simulink model "labcartpid_new"  (Simulink 10.2)
settings: Solver=FixedStepAuto  StartTime=0.0  StopTime=29  FixedStep=0.001  RelTol=1e-3
values from neighbouring files (symbols this model uses):
  X_MAX = 0.6    [5.1wksp_1.mat]
undefined symbols (not defined in the file or in its folder): HIL, qc_get_step_size
libraries: quarc_library x5, simulink_need_slupdate x1, simulink x1
settings Model: Creator=pcadm  LastModifiedBy=pcadm  ExtModeTrigDuration=15000
settings SolverCC: PositivePriorityOrder=on
settings DataIOCC: SaveFormat=Dataset  SignalLoggingSaveFormat=Dataset
settings DebuggingCC: UnderspecifiedInitializationDetection=Simplified  MergeDetectMultiDrivingBlocksExec=error  FcnCallInpInsideContextMsg=error  SFUnexpectedBacktrackingDiag=error  SFNoUnconditionalDefaultTransitionDiag=error  SFExecutionAtInitializationDiag=warning
settings HardwareCC: ProdBitPerPointer=64  ProdBitPerSizeT=64  ProdBitPerPtrDiffT=64  ProdLargestAtomicFloat=Float  ProdIntDivRoundTo=Zero  ProdEndianess=LittleEndian  ProdWordSize=64  ProdHWDeviceType=Intel->x86-64 (Windows64)
settings ModelReferenceCC: PropagateSignalLabelsOutOfModel=on
settings RTWCC: Description=QUARC Win64 Target  SystemTargetFile=quarc_win64.tlc  TemplateMakefile=quarc_default_tmf
settings STFCustomTargetCC: TargetPreCompLibLocation=C:\PROGRA~3\QUARC\lib\2020b\win64\release  TargetLangStandard=C99 (ISO)  ConcurrentExecutionCompliant=on  SystemTargetFile=quarc_win64.tlc
settings GRTTargetCC: TargetPreCompLibLocation=C:\PROGRA~3\QUARC\lib\2020b\win64\release  TargetLangStandard=C99 (ISO)  ParMdlRefBuildCompliant=off  CompOptLevelCompliant=off  MatFileLogging=off  CPPClassGenCompliant=off  UseToolchainInfoCompliant=off  ExtMode=on  ExtModeMexFile=quarc_comm
settings ConfigComp: CovMetricSettings=dswe  CovSaveCumulativeToWorkspaceVar=off  CovSaveSingleToWorkspaceVar=off  CovExternalEMLEnable=on

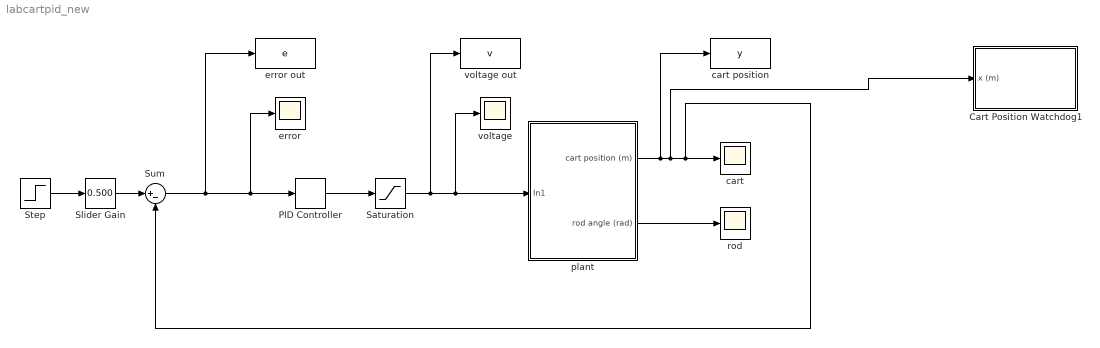
== system labcartpid_new ==
  Cart Position Watchdog1 : Subsystem  TreatAsAtomicUnit=on
  PID Controller : simulink_need_slupdate/PID Controller  P=80  I=2  D=10
  Saturation : Saturate  UpperLimit=6  LowerLimit=-6
  Slider Gain : simulink/Math Operations/Slider Gain  gain=0.500  low=-0.2  high=0.5
  Step : Step  Time=0  After=1.0  SampleTime=0
  Sum : Sum  Inputs=|+-
  cart : Scope
  cart position : ToWorkspace  VariableName=y  SaveFormat=Structure With Time  SampleTime=-1
  error : Scope
  error out : ToWorkspace  VariableName=e  SaveFormat=Structure  SampleTime=-1
  plant : Subsystem
  rod : Scope
  voltage : Scope
  voltage out : ToWorkspace  VariableName=v  SaveFormat=Structure  SampleTime=-1
  wires:
  Slider Gain/1 -> Sum/1
  Saturation/1 -> voltage out/1, plant/1(In1), voltage/1
  PID Controller/1 -> Saturation/1
  Sum/1 -> error/1, PID Controller/1, error out/1
  plant/1(cart position (m)) -> cart position/1, Cart Position Watchdog1/1(x (m)), cart/1, Sum/2
  Step/1 -> Slider Gain/1
  plant/2(rod angle (rad)) -> rod/1

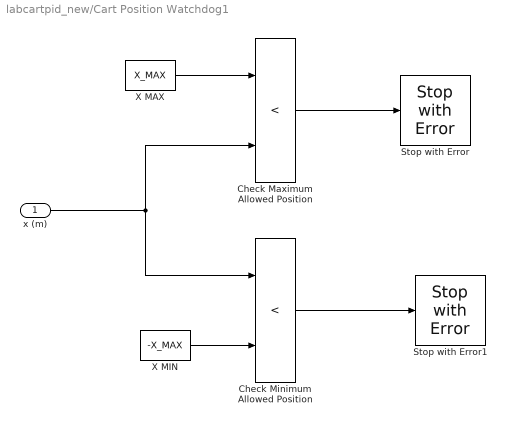
== system labcartpid_new/Cart Position Watchdog1 ==
  x (m) : Inport
  Check Maximum Allowed Position : RelationalOperator  Operator=<  RndMeth=Nearest  InputSameDT=on
  Check Minimum Allowed Position : RelationalOperator  Operator=<  RndMeth=Nearest  InputSameDT=on
  Stop with Error : quarc_library/Sinks/Error Handling/Stop with Error  message_type=Fixed error message  message=Maximum Limit Reached
      settings: AttributesFormatString="\"%<message>\""  SourceProductName=QUARC Targets
  Stop with Error1 : quarc_library/Sinks/Error Handling/Stop with Error  message_type=Fixed error message  message=Minimum Limit Reached
      settings: AttributesFormatString="\"%<message>\""  SourceProductName=QUARC Targets
  X MAX : Constant  Value=X_MAX
  X MIN : Constant  Value=-X_MAX
  wires:
  Check Maximum Allowed Position/1 -> Stop with Error/1
  x (m)/1 -> Check Minimum Allowed Position/1, Check Maximum Allowed Position/2
  X MIN/1 -> Check Minimum Allowed Position/2
  Check Minimum Allowed Position/1 -> Stop with Error1/1
  X MAX/1 -> Check Maximum Allowed Position/1

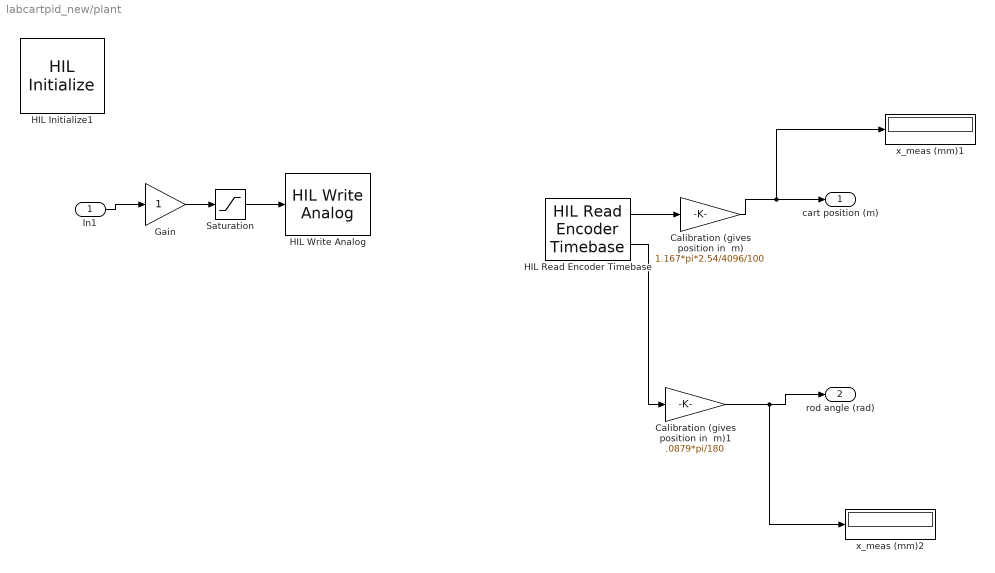
== system labcartpid_new/plant ==
  In1 : Inport
  Calibration (gives position in  m) : Gain  Gain=1.167*pi*2.54/4096/100  SaturateOnIntegerOverflow=on  OutDataTypeStr=Inherit: Same as input  ParamDataTypeStr=Inherit: Same as input
  Calibration (gives position in  m)1 : Gain  Gain=.0879*pi/180  SaturateOnIntegerOverflow=on  OutDataTypeStr=Inherit: Same as input  ParamDataTypeStr=Inherit: Same as input
  Gain : Gain  SaturateOnIntegerOverflow=on  OutDataTypeStr=Inherit: Same as input  ParamDataTypeStr=Inherit: Same as input
  HIL Initialize1 : quarc_library/Data Acquisition/Generic/Configuration/HIL Initialize  object_name=HIL-1  board_type=q4  board_number=0  board_options=""  exclusive=off  active=off  hardware_clocks=[0:1]  clock_modes=[0 0]  initial_clock_frequencies=[]  set_clock_params_at_start=on  set_clock_params_at_switch_in=off  set_clock_frequencies_at_start=off  set_clock_frequencies_at_switch_in=off  analog_input_channels=[0:3]  analog_input_configurations=[]  analog_input_maximums=10  analog_input_minimums=-10  set_analog_input_params_at_start=off  set_analog_input_params_at_switch_in=off  analog_output_channels=[0:3]  analog_output_maximums=[10]  analog_output_minimums=[-10]  initial_analog_outputs=[0]  final_analog_outputs=[0]  watchdog_analog_outputs=0  set_analog_output_params_at_start=on  set_analog_output_params_at_switch_in=off  set_analog_outputs_at_start=on  set_analog_outputs_at_switch_in=off  set_analog_outputs_at_terminate=on  set_analog_outputs_at_switch_out=off  set_analog_outputs_on_watchdog=off  digital_input_channels=[8:15]  digital_output_channels=[0:7]  digital_output_configuration=[]  initial_digital_outputs=[0]  final_digital_outputs=[0]  watchdog_digital_outputs=[2]  set_digital_output_params_at_start=off  set_digital_output_params_at_switch_in=off  set_digital_outputs_at_start=on  set_digital_outputs_at_switch_in=off  set_digital_outputs_at_terminate=on  set_digital_outputs_at_switch_out=off  set_digital_outputs_on_watchdog=off  encoder_channels=[0:3]  quadrature=[4]  encoder_filter_frequency=(1/60e-9)/1  initial_encoder_counts=[0]  set_encoder_params_at_start=on  set_encoder_params_at_switch_in=off  set_encoder_counts_at_start=on  set_encoder_counts_at_switch_in=off  pwm_channels=[]  pwm_modes=[0]  pwm_frequency=(1/60e-9)/1024  pwm_configuration=[]  pwm_alignment=[]  pwm_polarity=[]  pwm_leading_deadband=[]  pwm_trailing_deadband=[]  initial_pwm_outputs=[0]  final_pwm_outputs=[0]  watchdog_pwm_outputs=[]  set_pwm_params_at_start=on  set_pwm_params_at_switch_in=off  set_pwm_outputs_at_start=on  set_pwm_outputs_at_switch_in=off  set_pwm_outputs_at_terminate=on  set_pwm_outputs_at_switch_out=off  set_pwm_outputs_on_watchdog=off  other_output_channels=[]  initial_other_outputs=[]  final_other_outputs=[]  watchdog_other_outputs=[]  set_other_outputs_at_start=off  set_other_outputs_at_switch_in=off  set_other_outputs_at_terminate=off  set_other_outputs_at_switch_out=off  set_other_outputs_on_watchdog=off
  HIL Read Encoder Timebase : quarc_library/Data Acquisition/Generic/Timebases/HIL Read Encoder Timebase  object_name=HIL-1  clock=1  channels=[0,1]  active=on  vector_output=off  data_type_mode=Inherit via back propagation  data_type=double  overflow_mode=Error on overflow  samples_in_buffer=max(ceil(1/qc_get_step_size), 1)
  HIL Write Analog : quarc_library/Data Acquisition/Generic/Immediate I//O/HIL Write Analog  object_name=HIL-1  channels=0  sample_time=-1  active=off  vector_input=on
  Saturation : Saturate  UpperLimit=6  LowerLimit=-6
  x_meas (mm)1 : Display
      settings: Decimation=100
  x_meas (mm)2 : Display
      settings: Decimation=100
  cart position (m) : Outport
  rod angle (rad) : Outport  Port=2
  wires:
  In1/1 -> Gain/1
  HIL Read Encoder Timebase/1 -> Calibration (gives position in  m)/1
  Calibration (gives position in  m)/1 -> x_meas (mm)1/1, cart position (m)/1
  Saturation/1 -> HIL Write Analog/1
  HIL Read Encoder Timebase/2 -> Calibration (gives position in  m)1/1
  Gain/1 -> Saturation/1
  Calibration (gives position in  m)1/1 -> x_meas (mm)2/1, rod angle (rad)/1
